simulink library "nonameslib"  (R2020a)
settings: Solver=VariableStepAuto  StartTime=0.0  StopTime=10.0  RelTol=1e-3
libraries: $bdroot x1
settings Model: Creator=lowlimb  LastModifiedBy=lowlimb

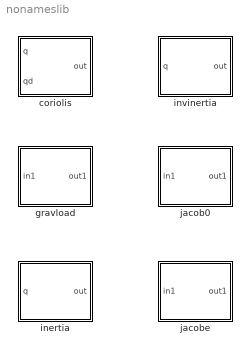
== system nonameslib ==
  coriolis : Subsystem
  gravload : MATLAB Function  TreatAsAtomicUnit=on
  inertia : Subsystem
  invinertia : Subsystem
  jacob0 : MATLAB Function  TreatAsAtomicUnit=on
  jacobe : MATLAB Function  TreatAsAtomicUnit=on

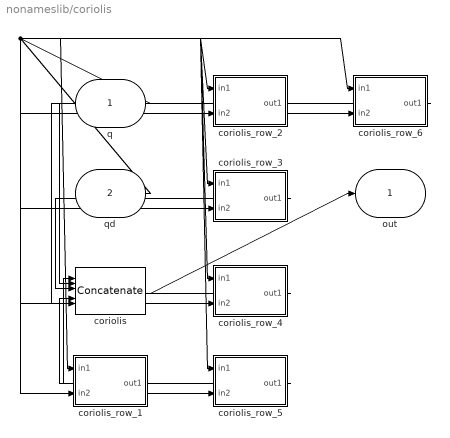
== system nonameslib/coriolis ==
  q : Inport
  qd : Inport  Port=2
  coriolis : Concatenate  NumInputs=6  Mode=Multidimensional array
  coriolis_row_1 : MATLAB Function  TreatAsAtomicUnit=on
  coriolis_row_2 : MATLAB Function  TreatAsAtomicUnit=on
  coriolis_row_3 : MATLAB Function  TreatAsAtomicUnit=on
  coriolis_row_4 : MATLAB Function  TreatAsAtomicUnit=on
  coriolis_row_5 : MATLAB Function  TreatAsAtomicUnit=on
  coriolis_row_6 : MATLAB Function  TreatAsAtomicUnit=on
  out : Outport
  wires:
  coriolis/1 -> out/1
  coriolis_row_1/1(out1) -> coriolis/1
  q/1 -> coriolis_row_1/1(in1), coriolis_row_2/1(in1), coriolis_row_3/1(in1), coriolis_row_4/1(in1), coriolis_row_5/1(in1), coriolis_row_6/1(in1)
  qd/1 -> coriolis_row_1/2(in2), coriolis_row_2/2(in2), coriolis_row_3/2(in2), coriolis_row_4/2(in2), coriolis_row_5/2(in2), coriolis_row_6/2(in2)
  coriolis_row_2/1(out1) -> coriolis/2
  coriolis_row_3/1(out1) -> coriolis/3
  coriolis_row_4/1(out1) -> coriolis/4
  coriolis_row_5/1(out1) -> coriolis/5
  coriolis_row_6/1(out1) -> coriolis/6

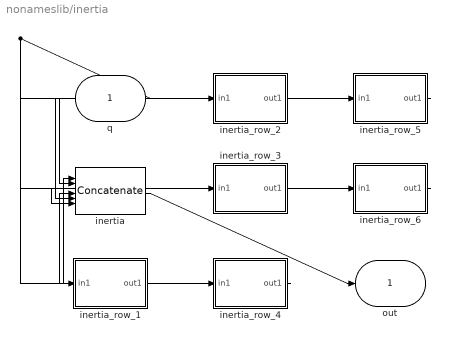
== system nonameslib/inertia ==
  q : Inport
  inertia : Concatenate  NumInputs=6  Mode=Multidimensional array
  inertia_row_1 : MATLAB Function  TreatAsAtomicUnit=on
  inertia_row_2 : MATLAB Function  TreatAsAtomicUnit=on
  inertia_row_3 : MATLAB Function  TreatAsAtomicUnit=on
  inertia_row_4 : MATLAB Function  TreatAsAtomicUnit=on
  inertia_row_5 : MATLAB Function  TreatAsAtomicUnit=on
  inertia_row_6 : MATLAB Function  TreatAsAtomicUnit=on
  out : Outport
  wires:
  inertia/1 -> out/1
  inertia_row_1/1(out1) -> inertia/1
  q/1 -> inertia_row_1/1(in1), inertia_row_2/1(in1), inertia_row_3/1(in1), inertia_row_4/1(in1), inertia_row_5/1(in1), inertia_row_6/1(in1)
  inertia_row_2/1(out1) -> inertia/2
  inertia_row_3/1(out1) -> inertia/3
  inertia_row_4/1(out1) -> inertia/4
  inertia_row_5/1(out1) -> inertia/5
  inertia_row_6/1(out1) -> inertia/6

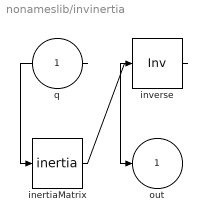
== system nonameslib/invinertia ==
  q : Inport
  inertiaMatrix : $bdroot/inertia  SystemSampleTime=-1  Latency=0  AutoFrameSizeCalculation=off
  inverse : Product  Inputs=/  Multiplication=Matrix(*)
  out : Outport
  wires:
  q/1 -> inertiaMatrix/1
  inertiaMatrix/1 -> inverse/1
  inverse/1 -> out/1

== matlab function nonameslib/inertia/inertia_row_6 ==
  data: in1 input; out1 output
function out1 = inertia_row_6(in1)
%#codegen

%    This function was generated by the Symbolic Math Toolbox version 8.5.
%    25-Apr-2020 14:33:48

q2 = in1(:,2);
q3 = in1(:,3);
q4 = in1(:,4);
q5 = in1(:,5);
q6 = in1(:,6);
t2 = cos(q3);
t3 = cos(q4);
t4 = cos(q5);
t5 = cos(q6);
t6 = sin(q3);
t7 = sin(q4);
t8 = sin(q5);
t9 = sin(q6);
t10 = t4.*t5.*1.365e-1;
t11 = t4.*t5.*5.46e-2;
t12 = t4.*t9.*1.365e-1;
t13 = t5.*t8.*1.365e-1;
t14 = t8.*t9.*1.365e-1;
t15 = t8.*t9.*5.46e-2;
t18 = t5.*3.549e-2;
t16 = -t14;
t17 = -t15;
t19 = t12+t13;
t20 = t10+t16;
t21 = t3.*t19;
t22 = t7.*t19;
t26 = t11+t17+t18+1.7745e-2;
t23 = t3.*t20;
t24 = t7.*t20;
t25 = -t22;
t27 = t21+t24;
t28 = t23+t25;
t31 = t2.*(t22-t23).*(-2.0./5.0);
t29 = t6.*t27.*(2.0./5.0);
t30 = -t29;
out1 = [t26+t30+t31-cos(q2).*(t6.*t27+t2.*(t22-t23)).*(4.3e+1./1.0e+2)-sin(q2).*(t2.*t27-t6.*(t22-t23)).*(4.3e+1./1.0e+2),t26+t30+t31,t26,t26,t18+1.7745e-2,1.7745e-2];

== matlab function nonameslib/coriolis/coriolis_row_6 ==
  data: in1 input; out1 output; in2 input
function out1 = coriolis_row_6(in1,in2)
%#codegen

%    This function was generated by the Symbolic Math Toolbox version 8.5.
%    28-Apr-2020 10:49:10

q2 = in1(:,2);
q3 = in1(:,3);
q4 = in1(:,4);
q5 = in1(:,5);
q6 = in1(:,6);
qd1 = in2(:,1);
qd2 = in2(:,2);
qd3 = in2(:,3);
qd4 = in2(:,4);
qd5 = in2(:,5);
t2 = sin(q6);
t3 = q5+q6;
t4 = sin(t3);
t5 = q3+q4+t3;
t11 = qd1.*t2.*3.549e-2;
t12 = qd2.*t2.*3.549e-2;
t13 = qd3.*t2.*3.549e-2;
t14 = qd4.*t2.*3.549e-2;
t15 = qd5.*t2.*3.549e-2;
t6 = sin(t5);
t7 = qd1.*t4.*5.46e-2;
t8 = qd2.*t4.*5.46e-2;
t9 = qd3.*t4.*5.46e-2;
t10 = qd4.*t4.*5.46e-2;
t16 = qd1.*t6.*5.46e-2;
t17 = qd2.*t6.*5.46e-2;
t18 = t7+t8+t9+t10+t11+t12+t13+t14+t15;
out1 = [t16+t17+t18+qd1.*sin(q2+t5).*5.8695e-2,t16+t17+t18,t18,t18,t2.*(qd1+qd2+qd3+qd4+qd5).*3.549e-2,0.0];

== matlab function nonameslib/inertia/inertia_row_1 ==
  data: in1 input; out1 output
function out1 = inertia_row_1(in1)
%#codegen

%    This function was generated by the Symbolic Math Toolbox version 8.5.
%    25-Apr-2020 14:04:22

q2 = in1(:,2);
q3 = in1(:,3);
q4 = in1(:,4);
q5 = in1(:,5);
q6 = in1(:,6);
t2 = cos(q2);
t3 = cos(q3);
t4 = cos(q4);
t5 = cos(q5);
t6 = cos(q6);
t7 = sin(q2);
t8 = sin(q3);
t9 = sin(q4);
t10 = sin(q5);
t11 = sin(q6);
t12 = t2.*(4.3e+1./1.0e+2);
t13 = t3.*t7.*(4.3e+1./1.0e+2);
t14 = t7.*t8.*(4.3e+1./1.0e+2);
t18 = t3.*t7.*1.75139e+1;
t19 = t7.*t8.*1.75139e+1;
t20 = t2.*7.68453e-1;
t22 = t7.*t8.*5.079031;
t15 = t12+2.0./5.0;
t23 = -t22;
t16 = t3.*t15;
t17 = t8.*t15;
t21 = -t16;
t24 = t16.*4.073e+1;
t25 = t17.*4.073e+1;
t27 = t13+t17;
t28 = t16.*1.18117e+1;
t26 = -t24;
t29 = t14+t21;
t30 = t4.*t27;
t31 = t9.*t27;
t32 = t4.*t29;
t33 = t9.*t29;
t35 = t30.*(7.77e+2./1.0e+2);
t36 = t31.*(7.77e+2./1.0e+2);
t40 = t31.*1.3209;
t34 = -t33;
t37 = -t35;
t38 = t32.*(7.77e+2./1.0e+2);
t39 = t33.*(7.77e+2./1.0e+2);
t41 = -t40;
t42 = t32.*1.3209;
t45 = t31+t32-2.0./5.0;
t43 = -t42;
t44 = t30+t34;
t48 = t5.*t45;
t49 = t10.*t45;
t46 = t5.*t44;
t47 = t10.*t44;
t50 = -t49;
t54 = t48.*(8.8e+1./2.5e+1);
t55 = t49.*(8.8e+1./2.5e+1);
t58 = t48.*(4.18e+2./6.25e+2);
t51 = t46.*(8.8e+1./2.5e+1);
t52 = t47.*(8.8e+1./2.5e+1);
t56 = t47.*(4.18e+2./6.25e+2);
t59 = -t58;
t60 = t46+t50;
t61 = t47+t48-1.3e+1./5.0e+1;
t53 = -t51;
t57 = -t56;
t62 = t11.*t60.*(2.1e+1./2.0e+1);
t63 = t6.*t60.*(2.1e+1./2.0e+1);
t65 = t11.*t60.*1.365e-1;
t66 = t11.*t61.*(2.1e+1./2.0e+1);
t68 = t6.*t61.*(2.1e+1./2.0e+1);
t69 = t6.*t61.*1.365e-1;
t64 = -t63;
t67 = -t65;
t70 = -t69;
t72 = -t6.*(t63-t66);
t73 = -t11.*(t63-t66);
t74 = t62+t68-1.365e-1;
t75 = t11.*(t63-t66).*(-1.3e+1./5.0e+1);
t76 = t11.*(t63-t66).*(1.3e+1./5.0e+1);
t71 = t64+t66;
t77 = t6.*t74;
t78 = t11.*t74;
t79 = -t78;
t80 = t77.*(1.3e+1./5.0e+1);
t83 = -t5.*(t51-t55+t78+t6.*(t63-t66));
t84 = -t10.*(t51-t55+t78+t6.*(t63-t66));
t85 = t10.*(t51-t55+t78+t6.*(t63-t66)).*(-2.0./5.0);
t86 = t52+t54+t73+t77-4.18e+2./6.25e+2;
t87 = t10.*(t51-t55+t78+t6.*(t63-t66)).*(2.0./5.0);
t81 = -t80;
t82 = t53+t55+t72+t79;
t88 = t5.*t86;
t89 = t10.*t86;
t90 = -t89;
t91 = t88.*(2.0./5.0);
t94 = -t9.*(t35-t39+t89+t5.*(t51-t55+t78+t6.*(t63-t66)));
t95 = -t4.*(t35-t39+t89+t5.*(t51-t55+t78+t6.*(t63-t66)));
t96 = t4.*(t35-t39+t89+t5.*(t51-t55+t78+t6.*(t63-t66)));
t97 = t36+t38+t84+t88-1.3209;
t92 = -t91;
t93 = t37+t39+t83+t90;
t98 = t9.*t97;
t99 = t4.*t97;
t100 = t18+t25+t96+t98;
t102 = t19+t26+t94+t99-1.18117e+1;
t103 = t3.*(-t19+t24-t99+t9.*(t35-t39+t89+t5.*(t51-t55+t78+t6.*(t63-t66)))+1.18117e+1).*(-2.0./5.0);
t104 = t3.*(-t19+t24-t99+t9.*(t35-t39+t89+t5.*(t51-t55+t78+t6.*(t63-t66)))+1.18117e+1).*(2.0./5.0);
t101 = t8.*t100.*(2.0./5.0);
out1 = [t20+t23+t28+t41+t43+t57+t59+t67+t70+t76+t81+t87+t92+t101+t104+t7.*(t7.*3.3411+t3.*t100-t8.*(-t19+t24-t99+t9.*(t35-t39+t89+t5.*(t51-t55+t78+t6.*(t63-t66)))+1.18117e+1)).*(4.3e+1./1.0e+2)+t12.*(t2.*3.3411+t8.*t100+t3.*(-t19+t24-t99+t9.*(t35-t39+t89+t5.*(t51-t55+t78+t6.*(t63-t66)))+1.18117e+1)+1.7871)+4.408548,t20+t23+t28+t41+t43+t57+t59+t67+t70+t76+t81+t87+t92+t101+t104+4.205796,t23+t28+t41+t43+t57+t59+t67+t70+t76+t81+t87+t92+3.794763,t41+t43+t57+t59+t67+t70+t76+t81+t87+t92+3.6937e-1,t57+t59+t67+t70+t76+t81+1.44817e-1,t67+t70+1.7745e-2];

== matlab function nonameslib/inertia/inertia_row_3 ==
  data: in1 input; out1 output
function out1 = inertia_row_3(in1)
%#codegen

%    This function was generated by the Symbolic Math Toolbox version 8.5.
%    25-Apr-2020 14:32:44

q2 = in1(:,2);
q3 = in1(:,3);
q4 = in1(:,4);
q5 = in1(:,5);
q6 = in1(:,6);
t2 = cos(q3);
t3 = cos(q4);
t4 = cos(q5);
t5 = cos(q6);
t6 = sin(q3);
t7 = sin(q4);
t8 = sin(q5);
t9 = sin(q6);
t10 = t4.*(2.0./5.0);
t11 = t5.*t8.*(2.1e+1./5.0e+1);
t12 = t8.*t9.*(2.1e+1./5.0e+1);
t13 = t4.*(1.76e+2./1.25e+2);
t14 = t8.*(1.76e+2./1.25e+2);
t16 = t4.*2.6752e-1;
t18 = t8.*t9.*5.46e-2;
t15 = -t12;
t17 = t10+1.3e+1./5.0e+1;
t19 = -t18;
t20 = t5.*t17.*(2.1e+1./2.0e+1);
t21 = t9.*t17.*(2.1e+1./2.0e+1);
t22 = t5.*t17.*1.365e-1;
t23 = t11+t21;
t27 = t15+t20+1.365e-1;
t24 = t5.*t23;
t25 = t9.*t23;
t28 = t5.*t27;
t29 = t9.*t27;
t26 = t25.*(1.3e+1./5.0e+1);
t30 = -t29;
t31 = t28.*(1.3e+1./5.0e+1);
t35 = t13+t25+t28+4.18e+2./6.25e+2;
t32 = t14+t24+t30;
t37 = t4.*t35;
t38 = t8.*t35;
t40 = t10.*t35;
t33 = t4.*t32;
t34 = t8.*t32;
t39 = -t38;
t36 = t34.*(2.0./5.0);
t41 = t33+t39;
t44 = t34+t37+1.3209;
t42 = t3.*t41;
t43 = t7.*t41;
t45 = t3.*t44;
t46 = t7.*t44;
t47 = -t46;
t50 = t43+t45+1.18117e+1;
t48 = t42+t47;
t51 = t2.*t50.*(2.0./5.0);
t49 = t6.*t48.*(2.0./5.0);
out1 = [t16+t19+t22+t26+t31+t36+t40+t49+t51+cos(q2).*(t2.*t50+t6.*t48).*(4.3e+1./1.0e+2)+sin(q2).*(t2.*t48-t6.*t50).*(4.3e+1./1.0e+2)+3.794763,t16+t19+t22+t26+t31+t36+t40+t49+t51+3.794763,t16+t19+t22+t26+t31+t36+t40+3.794763,t16+t19+t22+t26+t31+t36+t40+3.6937e-1,t16+t19+t22+t26+t31+1.44817e-1,t19+t22+1.7745e-2];

== matlab function nonameslib/inertia/inertia_row_4 ==
  data: in1 input; out1 output
function out1 = inertia_row_4(in1)
%#codegen

%    This function was generated by the Symbolic Math Toolbox version 8.5.
%    25-Apr-2020 14:33:40

q2 = in1(:,2);
q3 = in1(:,3);
q4 = in1(:,4);
q5 = in1(:,5);
q6 = in1(:,6);
t2 = cos(q3);
t3 = cos(q4);
t4 = cos(q5);
t5 = cos(q6);
t6 = sin(q3);
t7 = sin(q4);
t8 = sin(q5);
t9 = sin(q6);
t10 = t4.*(2.0./5.0);
t11 = t5.*t8.*(2.1e+1./5.0e+1);
t12 = t8.*t9.*(2.1e+1./5.0e+1);
t13 = t4.*(1.76e+2./1.25e+2);
t14 = t8.*(1.76e+2./1.25e+2);
t16 = t4.*2.6752e-1;
t18 = t8.*t9.*5.46e-2;
t15 = -t12;
t17 = t10+1.3e+1./5.0e+1;
t19 = -t18;
t20 = t5.*t17.*(2.1e+1./2.0e+1);
t21 = t9.*t17.*(2.1e+1./2.0e+1);
t22 = t5.*t17.*1.365e-1;
t23 = t11+t21;
t27 = t15+t20+1.365e-1;
t24 = t5.*t23;
t25 = t9.*t23;
t28 = t5.*t27;
t29 = t9.*t27;
t26 = t25.*(1.3e+1./5.0e+1);
t30 = -t29;
t31 = t28.*(1.3e+1./5.0e+1);
t35 = t13+t25+t28+4.18e+2./6.25e+2;
t32 = t14+t24+t30;
t37 = t4.*t35;
t38 = t8.*t35;
t40 = t10.*t35;
t33 = t4.*t32;
t34 = t8.*t32;
t39 = -t38;
t36 = t34.*(2.0./5.0);
t41 = t33+t39;
t44 = t34+t37+1.3209;
t42 = t3.*t41;
t43 = t7.*t41;
t45 = t3.*t44;
t46 = t7.*t44;
t48 = t16+t19+t22+t26+t31+t36+t40+3.6937e-1;
t47 = -t46;
t49 = t43+t45;
t50 = t42+t47;
t51 = t2.*t49.*(2.0./5.0);
t52 = t6.*t50.*(2.0./5.0);
out1 = [t48+t51+t52+cos(q2).*(t2.*t49+t6.*t50).*(4.3e+1./1.0e+2)+sin(q2).*(t2.*t50-t6.*t49).*(4.3e+1./1.0e+2),t48+t51+t52,t48,t48,t16+t19+t22+t26+t31+1.44817e-1,t19+t22+1.7745e-2];

== matlab function nonameslib/inertia/inertia_row_5 ==
  data: in1 input; out1 output
function out1 = inertia_row_5(in1)
%#codegen

%    This function was generated by the Symbolic Math Toolbox version 8.5.
%    25-Apr-2020 14:33:47

q2 = in1(:,2);
q3 = in1(:,3);
q4 = in1(:,4);
q5 = in1(:,5);
q6 = in1(:,6);
t2 = cos(q3);
t3 = cos(q4);
t4 = cos(q5);
t5 = cos(q6);
t6 = sin(q3);
t7 = sin(q4);
t8 = sin(q5);
t9 = sin(q6);
t10 = t9.^2;
t11 = t5.*(2.73e+2./1.0e+3);
t14 = t5.*3.549e-2;
t12 = t9.*t11;
t13 = t10.*(2.73e+2./1.0e+3);
t15 = t10.*7.098e-2;
t16 = t11+1.365e-1;
t17 = t5.*t16;
t18 = t9.*t16;
t19 = -t18;
t20 = t17.*(1.3e+1./5.0e+1);
t22 = -t4.*(t18-t5.*t9.*(2.73e+2./1.0e+3));
t23 = -t8.*(t18-t5.*t9.*(2.73e+2./1.0e+3));
t24 = t4.*(t18-t5.*t9.*(2.73e+2./1.0e+3));
t25 = t8.*(t18-t5.*t9.*(2.73e+2./1.0e+3)).*(-2.0./5.0);
t26 = t13+t17+4.18e+2./6.25e+2;
t21 = t12+t19;
t27 = t8.*t26;
t28 = t4.*t26;
t29 = t28.*(2.0./5.0);
t30 = t23+t28;
t31 = t24+t27;
t32 = t3.*t30;
t33 = t7.*t30;
t34 = t3.*t31;
t35 = t7.*t31;
t37 = t14+t15+t20+t25+t29+1.44817e-1;
t36 = -t35;
t38 = t33+t34;
t39 = t32+t36;
t40 = t6.*t38.*(2.0./5.0);
t41 = -t40;
t42 = t2.*t39.*(2.0./5.0);
out1 = [t37+t41+t42+cos(q2).*(t2.*t39-t6.*t38).*(4.3e+1./1.0e+2)-sin(q2).*(t2.*t38+t6.*t39).*(4.3e+1./1.0e+2),t37+t41+t42,t37,t37,t14+t15+t20+1.44817e-1,t14+1.7745e-2];

== matlab function nonameslib/gravload ==
  data: in1 input; out1 output
function out1 = gravload(in1)
%#codegen

%    This function was generated by the Symbolic Math Toolbox version 8.5.
%    28-Apr-2020 10:48:14

q1 = in1(:,1);
q2 = in1(:,2);
q3 = in1(:,3);
q4 = in1(:,4);
q5 = in1(:,5);
q6 = in1(:,6);
t2 = cos(q1);
t3 = cos(q2);
t4 = cos(q3);
t5 = cos(q4);
t6 = cos(q5);
t7 = cos(q6);
t8 = sin(q1);
t9 = sin(q2);
t10 = sin(q3);
t11 = sin(q4);
t12 = sin(q5);
t13 = sin(q6);
t14 = t2.*t3.*(9.81e+2./1.0e+2);
t15 = t2.*t9.*(9.81e+2./1.0e+2);
t16 = t3.*t8.*(9.81e+2./1.0e+2);
t17 = t8.*t9.*(9.81e+2./1.0e+2);
t19 = t2.*t3.*1.7531451e+1;
t20 = t8.*t9.*1.7531451e+1;
t18 = -t17;
t21 = -t20;
t22 = t15+t16;
t23 = t14+t18;
t24 = t4.*t22;
t25 = t10.*t22;
t26 = t4.*t23;
t27 = t10.*t23;
t28 = -t25;
t29 = t24.*4.073e+1;
t30 = t25.*4.073e+1;
t34 = t25.*1.18117e+1;
t31 = t26.*4.073e+1;
t32 = t27.*4.073e+1;
t33 = -t30;
t35 = t26.*1.18117e+1;
t36 = -t34;
t37 = t24+t27;
t38 = t26+t28;
t41 = -t5.*(t25-t26);
t42 = -t11.*(t25-t26);
t47 = t5.*(t25-t26).*(-7.77e+2./1.0e+2);
t48 = t11.*(t25-t26).*(-7.77e+2./1.0e+2);
t51 = t5.*(t25-t26).*(-1.3209);
t39 = t5.*t37;
t40 = t11.*t37;
t43 = -t40;
t44 = t39.*(7.77e+2./1.0e+2);
t45 = t40.*(7.77e+2./1.0e+2);
t49 = t40.*1.3209;
t52 = t39+t42;
t56 = -t12.*(t40+t5.*(t25-t26));
t57 = -t6.*(t40+t5.*(t25-t26));
t58 = t6.*(t40+t5.*(t25-t26));
t61 = t12.*(t40+t5.*(t25-t26)).*(-8.8e+1./2.5e+1);
t46 = -t45;
t50 = -t49;
t53 = t41+t43;
t54 = t12.*t52;
t55 = t6.*t52;
t63 = t58.*(-8.8e+1./2.5e+1);
t65 = t58.*(8.8e+1./2.5e+1);
t66 = t58.*(-4.18e+2./6.25e+2);
t59 = t54.*(8.8e+1./2.5e+1);
t60 = t55.*(8.8e+1./2.5e+1);
t62 = t54.*(4.18e+2./6.25e+2);
t67 = t55+t56;
t68 = t54+t58;
t64 = -t62;
t69 = t7.*t67.*(2.1e+1./2.0e+1);
t70 = t13.*t67.*(2.1e+1./2.0e+1);
t71 = t7.*t68.*(2.1e+1./2.0e+1);
t72 = t13.*t68.*(2.1e+1./2.0e+1);
t74 = t13.*t67.*1.365e-1;
t76 = t7.*t68.*1.365e-1;
t73 = -t72;
t75 = -t74;
t77 = -t76;
t78 = t70+t71;
t79 = t69+t73;
t80 = t7.*t78;
t81 = t13.*t78;
t82 = t7.*t79;
t83 = t13.*t79;
t85 = t80.*(1.3e+1./5.0e+1);
t84 = -t83;
t86 = -t85;
t87 = t83.*(1.3e+1./5.0e+1);
t88 = t60+t61+t81+t82;
t89 = t59+t65+t80+t84;
t90 = t6.*t88;
t91 = t12.*t88;
t92 = t6.*t89;
t93 = t12.*t89;
t94 = t91.*(2.0./5.0);
t95 = -t92;
t96 = t92.*(2.0./5.0);
t98 = t44+t48+t90+t93;
t102 = -t5.*(t45-t91+t92+t5.*(t25-t26).*(7.77e+2./1.0e+2));
t103 = -t11.*(t45-t91+t92+t5.*(t25-t26).*(7.77e+2./1.0e+2));
t104 = t11.*(t45-t91+t92+t5.*(t25-t26).*(7.77e+2./1.0e+2));
t97 = -t96;
t99 = t46+t47+t91+t95;
t100 = t5.*t98;
t101 = t11.*t98;
t105 = t31+t33+t101+t102;
t106 = t29+t32+t100+t104;
t107 = t4.*(t30-t31-t101+t5.*(t45-t91+t92+t5.*(t25-t26).*(7.77e+2./1.0e+2))).*(-2.0./5.0);
t108 = t10.*t106.*(2.0./5.0);
out1 = [t2.*8.287488+t19+t21+t35+t36+t50+t51+t64+t66+t75+t77+t86+t87+t94+t97+t107+t108+t3.*(t2.*t3.*7.62237e+1-t8.*t9.*7.62237e+1+t10.*t106-t4.*(t30-t31-t101+t5.*(t45-t91+t92+t5.*(t25-t26).*(7.77e+2./1.0e+2)))).*(4.3e+1./1.0e+2)+t9.*(t2.*t9.*7.62237e+1+t3.*t8.*7.62237e+1+t4.*t106+t10.*(t30-t31-t101+t5.*(t45-t91+t92+t5.*(t25-t26).*(7.77e+2./1.0e+2)))).*(4.3e+1./1.0e+2),t19+t21+t35+t36+t50+t51+t64+t66+t75+t77+t86+t87+t94+t97+t107+t108,t35+t36+t50+t51+t64+t66+t75+t77+t86+t87+t94+t97,t50+t51+t64+t66+t75+t77+t86+t87+t94+t97,t64+t66+t75+t77+t86+t87,t75+t77];

== matlab function nonameslib/jacob0 ==
  data: in1 input; out1 output
function out1 = jacob0(in1)
%#codegen

%    This function was generated by the Symbolic Math Toolbox version 8.5.
%    28-Apr-2020 10:48:19

q1 = in1(:,1);
q2 = in1(:,2);
q3 = in1(:,3);
q4 = in1(:,4);
q5 = in1(:,5);
q6 = in1(:,6);
t2 = cos(q6);
t3 = sin(q6);
t4 = q5+q6;
t5 = cos(t4);
t6 = sin(t4);
t7 = q3+q4+t4;
t16 = t2.*(1.3e+1./5.0e+1);
t17 = t3.*(1.3e+1./5.0e+1);
t8 = cos(t7);
t9 = q2+t7;
t10 = sin(t7);
t14 = t5.*(2.0./5.0);
t15 = t6.*(2.0./5.0);
t11 = q1+t9;
t12 = sin(t9);
t13 = cos(t9);
t20 = t8.*(2.0./5.0);
t21 = t10.*(2.0./5.0);
t24 = t14+t16;
t25 = t15+t17;
t18 = cos(t11);
t19 = sin(t11);
t22 = t13.*(4.3e+1./1.0e+2);
t23 = t12.*(4.3e+1./1.0e+2);
t30 = t20+t24;
t31 = t21+t25;
t26 = t18.*t24;
t27 = t19.*t24;
t28 = t18.*t25;
t29 = t19.*t25;
t33 = t23+t31;
t34 = t22+t30;
t32 = -t27;
t35 = t26+t29;
t36 = t28+t32;
out1 = reshape([t18.*t33-t19.*t34,t18.*t34+t19.*t33,0.0,0.0,0.0,1.0,t18.*t31-t19.*t30,t18.*t30+t19.*t31,0.0,0.0,0.0,1.0,t36,t35,0.0,0.0,0.0,1.0,t36,t35,0.0,0.0,0.0,1.0,t2.*t19.*(-1.3e+1./5.0e+1)+t17.*t18,t16.*t18+t17.*t19,0.0,0.0,0.0,1.0,0.0,0.0,0.0,0.0,0.0,1.0],[6,6]);

== matlab function nonameslib/jacobe ==
  data: in1 input; out1 output
function out1 = jacobe(in1)
%#codegen

%    This function was generated by the Symbolic Math Toolbox version 8.5.
%    28-Apr-2020 10:48:19

q2 = in1(:,2);
q3 = in1(:,3);
q4 = in1(:,4);
q5 = in1(:,5);
q6 = in1(:,6);
t2 = cos(q6);
t3 = sin(q6);
t4 = q5+q6;
t5 = cos(t4);
t6 = sin(t4);
t7 = q3+q4+t4;
t13 = t2.*(1.3e+1./5.0e+1);
t14 = t3.*(1.3e+1./5.0e+1);
t8 = cos(t7);
t9 = q2+t7;
t10 = sin(t7);
t11 = t5.*(2.0./5.0);
t12 = t6.*(2.0./5.0);
t15 = t8.*(2.0./5.0);
t16 = t10.*(2.0./5.0);
t17 = t11+t13;
t18 = t12+t14;
out1 = reshape([t16+t18+sin(t9).*(4.3e+1./1.0e+2),t15+t17+cos(t9).*(4.3e+1./1.0e+2),0.0,0.0,0.0,1.0,t16+t18,t15+t17,0.0,0.0,0.0,1.0,t18,t17,0.0,0.0,0.0,1.0,t18,t17,0.0,0.0,0.0,1.0,t14,t13,0.0,0.0,0.0,1.0,0.0,0.0,0.0,0.0,0.0,1.0],[6,6]);

== matlab function nonameslib/coriolis/coriolis_row_1 ==
  data: in1 input; out1 output; in2 input
function out1 = coriolis_row_1(in1,in2)
%#codegen

%    This function was generated by the Symbolic Math Toolbox version 8.5.
%    28-Apr-2020 10:49:08

q2 = in1(:,2);
q3 = in1(:,3);
q4 = in1(:,4);
q5 = in1(:,5);
q6 = in1(:,6);
qd1 = in2(:,1);
qd2 = in2(:,2);
qd3 = in2(:,3);
qd4 = in2(:,4);
qd5 = in2(:,5);
qd6 = in2(:,6);
t2 = sin(q2);
t3 = sin(q3);
t4 = sin(q5);
t5 = sin(q6);
t6 = q2+q3;
t7 = q3+q4;
t8 = q5+q6;
t9 = q4+t6;
t10 = q5+t7;
t11 = sin(t6);
t12 = sin(t7);
t13 = sin(t8);
t15 = t7+t8;
t24 = qd5.*t4.*3.7672e-1;
t28 = qd6.*t5.*3.549e-2;
t36 = qd3.*t3.*4.72468;
t62 = qd2.*t2.*9.896493;
t14 = q5+t9;
t16 = sin(t9);
t17 = sin(t10);
t18 = t8+t9;
t20 = sin(t15);
t22 = qd5.*t13.*5.46e-2;
t23 = qd6.*t13.*5.46e-2;
t27 = -t24;
t35 = -t28;
t43 = qd1.*t12.*1.25956;
t44 = qd2.*t12.*1.25956;
t45 = qd3.*t12.*1.25956;
t46 = qd4.*t12.*1.25956;
t47 = -t36;
t68 = qd1.*t11.*5.079031;
t69 = qd2.*t11.*5.079031;
t70 = qd3.*t11.*5.079031;
t71 = -t62;
t19 = sin(t14);
t21 = sin(t18);
t25 = -t22;
t26 = -t23;
t29 = qd1.*t20.*5.46e-2;
t30 = qd2.*t20.*5.46e-2;
t31 = qd3.*t20.*5.46e-2;
t32 = qd4.*t20.*5.46e-2;
t33 = qd5.*t20.*5.46e-2;
t34 = qd6.*t20.*5.46e-2;
t48 = qd1.*t17.*3.7672e-1;
t49 = qd2.*t17.*3.7672e-1;
t50 = qd3.*t17.*3.7672e-1;
t51 = qd4.*t17.*3.7672e-1;
t52 = qd5.*t17.*3.7672e-1;
t53 = -t43;
t54 = -t44;
t55 = -t45;
t56 = -t46;
t83 = -t68;
t84 = -t69;
t85 = -t70;
t92 = qd1.*t16.*1.354027;
t93 = qd2.*t16.*1.354027;
t94 = qd3.*t16.*1.354027;
t95 = qd4.*t16.*1.354027;
t37 = -t29;
t38 = -t30;
t39 = -t31;
t40 = -t32;
t41 = -t33;
t42 = -t34;
t57 = -t48;
t58 = -t49;
t59 = -t50;
t60 = -t51;
t61 = -t52;
t63 = qd1.*t19.*4.04974e-1;
t64 = qd2.*t19.*4.04974e-1;
t65 = qd3.*t19.*4.04974e-1;
t66 = qd4.*t19.*4.04974e-1;
t67 = qd5.*t19.*4.04974e-1;
t72 = qd1.*t21.*5.8695e-2;
t73 = qd2.*t21.*5.8695e-2;
t74 = qd3.*t21.*5.8695e-2;
t75 = qd4.*t21.*5.8695e-2;
t76 = qd5.*t21.*5.8695e-2;
t77 = qd6.*t21.*5.8695e-2;
t96 = -t92;
t97 = -t93;
t98 = -t94;
t99 = -t95;
t78 = -t63;
t79 = -t64;
t80 = -t65;
t81 = -t66;
t82 = -t67;
t86 = -t72;
t87 = -t73;
t88 = -t74;
t89 = -t75;
t90 = -t76;
t91 = -t77;
out1 = [t25+t26+t27+t35+t39+t40+t41+t42+t47+t55+t56+t59+t60+t61+t71+t79+t80+t81+t82+t84+t85+t87+t88+t89+t90+t91+t97+t98+t99,t25+t26+t27+t35+t39+t40+t41+t42+t47+t55+t56+t59+t60+t61+t71+t78+t79+t80+t81+t82+t83+t84+t85+t86+t87+t88+t89+t90+t91+t96+t97+t98+t99-qd1.*t2.*9.896493,t25+t26+t27+t35+t37+t38+t39+t40+t41+t42+t47+t53+t54+t55+t56+t57+t58+t59+t60+t61+t78+t79+t80+t81+t82+t83+t84+t85+t86+t87+t88+t89+t90+t91+t96+t97+t98+t99-qd1.*t3.*4.72468-qd2.*t3.*4.72468,t25+t26+t27+t35+t37+t38+t39+t40+t41+t42+t53+t54+t55+t56+t57+t58+t59+t60+t61+t78+t79+t80+t81+t82+t86+t87+t88+t89+t90+t91+t96+t97+t98+t99,t25+t26+t27+t35+t37+t38+t39+t40+t41+t42+t57+t58+t59+t60+t61+t78+t79+t80+t81+t82+t86+t87+t88+t89+t90+t91-qd1.*t4.*3.7672e-1-qd2.*t4.*3.7672e-1-qd3.*t4.*3.7672e-1-qd4.*t4.*3.7672e-1-qd1.*t13.*5.46e-2-qd2.*t13.*5.46e-2-qd3.*t13.*5.46e-2-qd4.*t13.*5.46e-2,(t5.*2.6e+1+t13.*4.0e+1+t20.*4.0e+1+t21.*4.3e+1).*(qd1+qd2+qd3+qd4+qd5+qd6).*(-1.365e-3)];

== matlab function nonameslib/coriolis/coriolis_row_2 ==
  data: in1 input; out1 output; in2 input
function out1 = coriolis_row_2(in1,in2)
%#codegen

%    This function was generated by the Symbolic Math Toolbox version 8.5.
%    28-Apr-2020 10:49:09

q2 = in1(:,2);
q3 = in1(:,3);
q4 = in1(:,4);
q5 = in1(:,5);
q6 = in1(:,6);
qd1 = in2(:,1);
qd2 = in2(:,2);
qd3 = in2(:,3);
qd4 = in2(:,4);
qd5 = in2(:,5);
qd6 = in2(:,6);
t2 = sin(q3);
t3 = sin(q5);
t4 = sin(q6);
t5 = q3+q4;
t6 = q5+q6;
t7 = q5+t5;
t8 = sin(t5);
t9 = sin(t6);
t10 = t5+t6;
t15 = qd5.*t3.*3.7672e-1;
t19 = qd6.*t4.*3.549e-2;
t27 = qd3.*t2.*4.72468;
t11 = sin(t7);
t12 = sin(t10);
t13 = qd5.*t9.*5.46e-2;
t14 = qd6.*t9.*5.46e-2;
t18 = -t15;
t26 = -t19;
t34 = qd1.*t8.*1.25956;
t35 = qd2.*t8.*1.25956;
t36 = qd3.*t8.*1.25956;
t37 = qd4.*t8.*1.25956;
t38 = -t27;
t16 = -t13;
t17 = -t14;
t20 = qd1.*t12.*5.46e-2;
t21 = qd2.*t12.*5.46e-2;
t22 = qd3.*t12.*5.46e-2;
t23 = qd4.*t12.*5.46e-2;
t24 = qd5.*t12.*5.46e-2;
t25 = qd6.*t12.*5.46e-2;
t39 = qd1.*t11.*3.7672e-1;
t40 = qd2.*t11.*3.7672e-1;
t41 = qd3.*t11.*3.7672e-1;
t42 = qd4.*t11.*3.7672e-1;
t43 = qd5.*t11.*3.7672e-1;
t44 = -t34;
t45 = -t35;
t46 = -t36;
t47 = -t37;
t28 = -t20;
t29 = -t21;
t30 = -t22;
t31 = -t23;
t32 = -t24;
t33 = -t25;
t48 = -t39;
t49 = -t40;
t50 = -t41;
t51 = -t42;
t52 = -t43;
out1 = [t16+t17+t18+t26+t30+t31+t32+t33+t38+t46+t47+t50+t51+t52+qd1.*sin(q2+q3).*5.079031+qd1.*sin(q2+t5).*1.354027+qd1.*sin(q2+t7).*4.04974e-1+qd1.*sin(q2+t10).*5.8695e-2+qd1.*sin(q2).*9.896493,t16+t17+t18+t26+t30+t31+t32+t33+t38+t46+t47+t50+t51+t52,t16+t17+t18+t26+t28+t29+t30+t31+t32+t33+t38+t44+t45+t46+t47+t48+t49+t50+t51+t52-qd1.*t2.*4.72468-qd2.*t2.*4.72468,t16+t17+t18+t26+t28+t29+t30+t31+t32+t33+t44+t45+t46+t47+t48+t49+t50+t51+t52,t16+t17+t18+t26+t28+t29+t30+t31+t32+t33+t48+t49+t50+t51+t52-qd1.*t3.*3.7672e-1-qd2.*t3.*3.7672e-1-qd3.*t3.*3.7672e-1-qd4.*t3.*3.7672e-1-qd1.*t9.*5.46e-2-qd2.*t9.*5.46e-2-qd3.*t9.*5.46e-2-qd4.*t9.*5.46e-2,(t4.*1.3e+1+t9.*2.0e+1+t12.*2.0e+1).*(qd1+qd2+qd3+qd4+qd5+qd6).*(-2.73e-3)];

== matlab function nonameslib/inertia/inertia_row_2 ==
  data: in1 input; out1 output
function out1 = inertia_row_2(in1)
%#codegen

%    This function was generated by the Symbolic Math Toolbox version 8.5.
%    25-Apr-2020 14:31:48

q2 = in1(:,2);
q3 = in1(:,3);
q4 = in1(:,4);
q5 = in1(:,5);
q6 = in1(:,6);
t2 = cos(q3);
t3 = cos(q4);
t4 = cos(q5);
t5 = cos(q6);
t6 = sin(q3);
t7 = sin(q4);
t8 = sin(q5);
t9 = sin(q6);
t10 = t2.*t3.*(2.0./5.0);
t11 = t2.*t7.*(2.0./5.0);
t12 = t3.*t6.*(2.0./5.0);
t13 = t6.*t7.*(2.0./5.0);
t15 = t2.*1.6292e+1;
t16 = t6.*1.6292e+1;
t17 = t2.*t3.*(7.77e+2./2.5e+2);
t18 = t2.*t7.*(7.77e+2./2.5e+2);
t19 = t3.*t6.*(7.77e+2./2.5e+2);
t20 = t6.*t7.*(7.77e+2./2.5e+2);
t22 = t2.*4.72468;
t23 = t2.*t3.*5.2836e-1;
t24 = t6.*t7.*5.2836e-1;
t14 = -t13;
t21 = -t20;
t25 = -t24;
t26 = t11+t12;
t27 = t4.*t26;
t28 = t8.*t26;
t29 = t10+t14+2.0./5.0;
t30 = -t28;
t31 = t4.*t29;
t32 = t8.*t29;
t33 = t27.*(8.8e+1./2.5e+1);
t34 = t28.*(8.8e+1./2.5e+1);
t36 = t28.*(4.18e+2./6.25e+2);
t35 = -t34;
t37 = -t36;
t38 = t31.*(8.8e+1./2.5e+1);
t39 = t32.*(8.8e+1./2.5e+1);
t40 = t31.*(4.18e+2./6.25e+2);
t41 = t27+t32;
t42 = t30+t31+1.3e+1./5.0e+1;
t43 = t5.*t41.*(2.1e+1./2.0e+1);
t44 = t9.*t41.*(2.1e+1./2.0e+1);
t46 = t9.*t41.*1.365e-1;
t48 = t5.*t42.*(2.1e+1./2.0e+1);
t49 = t9.*t42.*(2.1e+1./2.0e+1);
t50 = t5.*t42.*1.365e-1;
t45 = -t44;
t47 = -t46;
t51 = t43+t49;
t52 = t9.*t51;
t53 = t5.*t51;
t55 = t45+t48+1.365e-1;
t54 = t52.*(1.3e+1./5.0e+1);
t56 = t9.*t55;
t57 = t5.*t55;
t58 = -t56;
t59 = t57.*(1.3e+1./5.0e+1);
t64 = t35+t38+t52+t57+4.18e+2./6.25e+2;
t60 = t33+t39+t53+t58;
t65 = t4.*t64;
t66 = t8.*t64;
t61 = t4.*t60;
t62 = t8.*t60;
t67 = -t66;
t68 = t65.*(2.0./5.0);
t63 = t62.*(2.0./5.0);
t69 = t18+t19+t61+t67;
t72 = t17+t21+t62+t65+1.3209;
t70 = t3.*t69;
t71 = t7.*t69;
t73 = t3.*t72;
t74 = t7.*t72;
t75 = -t74;
t78 = t15+t71+t73+1.18117e+1;
t76 = t16+t70+t75;
t79 = t2.*t78.*(2.0./5.0);
t77 = t6.*t76.*(2.0./5.0);
out1 = [t22+t23+t25+t37+t40+t47+t50+t54+t59+t63+t68+t77+t79+cos(q2).*(t2.*t78+t6.*t76+1.7871).*(4.3e+1./1.0e+2)+sin(q2).*(t2.*t76-t6.*t78).*(4.3e+1./1.0e+2)+4.205796,t22+t23+t25+t37+t40+t47+t50+t54+t59+t63+t68+t77+t79+4.205796,t22+t23+t25+t37+t40+t47+t50+t54+t59+t63+t68+3.794763,t23+t25+t37+t40+t47+t50+t54+t59+t63+t68+3.6937e-1,t37+t40+t47+t50+t54+t59+1.44817e-1,t47+t50+1.7745e-2];

== matlab function nonameslib/coriolis/coriolis_row_3 ==
  data: in1 input; out1 output; in2 input
function out1 = coriolis_row_3(in1,in2)
%#codegen

%    This function was generated by the Symbolic Math Toolbox version 8.5.
%    28-Apr-2020 10:49:09

q2 = in1(:,2);
q3 = in1(:,3);
q4 = in1(:,4);
q5 = in1(:,5);
q6 = in1(:,6);
qd1 = in2(:,1);
qd2 = in2(:,2);
qd3 = in2(:,3);
qd4 = in2(:,4);
qd5 = in2(:,5);
qd6 = in2(:,6);
t2 = sin(q3);
t3 = sin(q5);
t4 = sin(q6);
t5 = q3+q4;
t6 = q5+q6;
t7 = q5+t5;
t8 = sin(t5);
t9 = sin(t6);
t10 = t5+t6;
t15 = qd5.*t3.*3.7672e-1;
t19 = qd6.*t4.*3.549e-2;
t23 = qd1.*t2.*4.72468;
t24 = qd2.*t2.*4.72468;
t11 = sin(t7);
t12 = sin(t10);
t13 = qd5.*t9.*5.46e-2;
t14 = qd6.*t9.*5.46e-2;
t18 = -t15;
t22 = -t19;
t25 = qd1.*t8.*1.25956;
t26 = qd2.*t8.*1.25956;
t16 = -t13;
t17 = -t14;
t20 = qd1.*t12.*5.46e-2;
t21 = qd2.*t12.*5.46e-2;
t27 = qd1.*t11.*3.7672e-1;
t28 = qd2.*t11.*3.7672e-1;
t29 = t16+t17+t18+t22;
out1 = [t20+t21+t23+t24+t25+t26+t27+t28+t29+qd1.*sin(q2+q3).*5.079031+qd1.*sin(q2+t5).*1.354027+qd1.*sin(q2+t7).*4.04974e-1+qd1.*sin(q2+t10).*5.8695e-2,t20+t21+t23+t24+t25+t26+t27+t28+t29,t29,t29,t29-qd1.*t3.*3.7672e-1-qd2.*t3.*3.7672e-1-qd3.*t3.*3.7672e-1-qd4.*t3.*3.7672e-1-qd1.*t9.*5.46e-2-qd2.*t9.*5.46e-2-qd3.*t9.*5.46e-2-qd4.*t9.*5.46e-2,(t4.*1.3e+1+t9.*2.0e+1).*(qd1+qd2+qd3+qd4+qd5+qd6).*(-2.73e-3)];

== matlab function nonameslib/coriolis/coriolis_row_4 ==
  data: in1 input; out1 output; in2 input
function out1 = coriolis_row_4(in1,in2)
%#codegen

%    This function was generated by the Symbolic Math Toolbox version 8.5.
%    28-Apr-2020 10:49:10

q2 = in1(:,2);
q3 = in1(:,3);
q4 = in1(:,4);
q5 = in1(:,5);
q6 = in1(:,6);
qd1 = in2(:,1);
qd2 = in2(:,2);
qd3 = in2(:,3);
qd4 = in2(:,4);
qd5 = in2(:,5);
qd6 = in2(:,6);
t2 = sin(q5);
t3 = sin(q6);
t4 = q3+q4;
t5 = q5+q6;
t6 = q5+t4;
t7 = sin(t4);
t8 = sin(t5);
t9 = t4+t5;
t14 = qd5.*t2.*3.7672e-1;
t18 = qd6.*t3.*3.549e-2;
t10 = sin(t6);
t11 = sin(t9);
t12 = qd5.*t8.*5.46e-2;
t13 = qd6.*t8.*5.46e-2;
t17 = -t14;
t21 = -t18;
t22 = qd1.*t7.*1.25956;
t23 = qd2.*t7.*1.25956;
t15 = -t12;
t16 = -t13;
t19 = qd1.*t11.*5.46e-2;
t20 = qd2.*t11.*5.46e-2;
t24 = qd1.*t10.*3.7672e-1;
t25 = qd2.*t10.*3.7672e-1;
t26 = t15+t16+t17+t21;
out1 = [t19+t20+t22+t23+t24+t25+t26+qd1.*sin(q2+t4).*1.354027+qd1.*sin(q2+t6).*4.04974e-1+qd1.*sin(q2+t9).*5.8695e-2,t19+t20+t22+t23+t24+t25+t26,t26,t26,t26-qd1.*t2.*3.7672e-1-qd2.*t2.*3.7672e-1-qd3.*t2.*3.7672e-1-qd4.*t2.*3.7672e-1-qd1.*t8.*5.46e-2-qd2.*t8.*5.46e-2-qd3.*t8.*5.46e-2-qd4.*t8.*5.46e-2,(t3.*1.3e+1+t8.*2.0e+1).*(qd1+qd2+qd3+qd4+qd5+qd6).*(-2.73e-3)];

== matlab function nonameslib/coriolis/coriolis_row_5 ==
  data: in1 input; out1 output; in2 input
function out1 = coriolis_row_5(in1,in2)
%#codegen

%    This function was generated by the Symbolic Math Toolbox version 8.5.
%    28-Apr-2020 10:49:10

q2 = in1(:,2);
q3 = in1(:,3);
q4 = in1(:,4);
q5 = in1(:,5);
q6 = in1(:,6);
qd1 = in2(:,1);
qd2 = in2(:,2);
qd3 = in2(:,3);
qd4 = in2(:,4);
qd5 = in2(:,5);
qd6 = in2(:,6);
t2 = sin(q5);
t3 = sin(q6);
t4 = q5+q6;
t5 = q3+q4+q5;
t6 = sin(t4);
t7 = q3+q4+t4;
t8 = sin(t5);
t14 = qd1.*t2.*3.7672e-1;
t15 = qd2.*t2.*3.7672e-1;
t16 = qd3.*t2.*3.7672e-1;
t17 = qd4.*t2.*3.7672e-1;
t18 = qd6.*t3.*3.549e-2;
t9 = sin(t7);
t10 = qd1.*t6.*5.46e-2;
t11 = qd2.*t6.*5.46e-2;
t12 = qd3.*t6.*5.46e-2;
t13 = qd4.*t6.*5.46e-2;
t21 = -t18;
t22 = qd1.*t8.*3.7672e-1;
t23 = qd2.*t8.*3.7672e-1;
t19 = qd1.*t9.*5.46e-2;
t20 = qd2.*t9.*5.46e-2;
t24 = t10+t11+t12+t13+t14+t15+t16+t17+t21;
out1 = [t19+t20+t22+t23+t24+qd1.*sin(q2+t5).*4.04974e-1+qd1.*sin(q2+t7).*5.8695e-2,t19+t20+t22+t23+t24,t24,t24,t21,t3.*(qd1+qd2+qd3+qd4+qd5+qd6).*(-3.549e-2)];
